simulink model "practika"  (R2024a)
settings: Solver=VariableStepAuto  StartTime=0.0  StopTime=15.0  RelTol=1e-3
model workspace (MAT data in the model file):
  diff_x = 0
  int_x = 0
  x = [1; 0]
  x1 = [-2; 0]
settings Model: Creator=Кирилл  LastModifiedBy=Анастасия
settings OptimizationCC: ReuseModelBlockBuffer=off
settings RTWCC: GPUComputeCapability=3.5

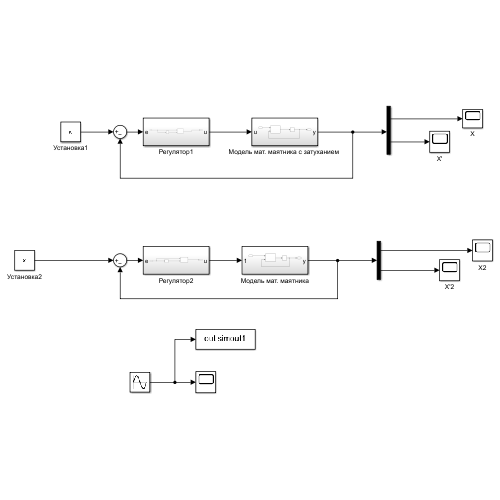
[thumbnail: Simulink's stored preview of the top-level diagram]
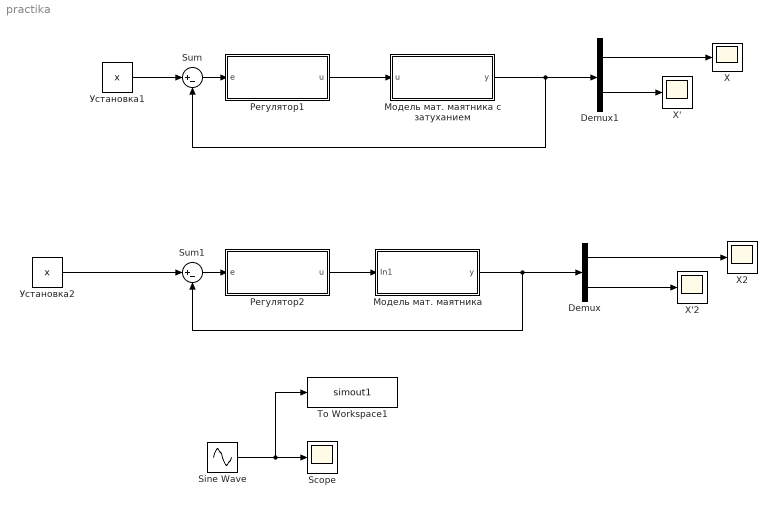
== system practika ==
  Demux : Demux  Outputs=2
  Demux1 : Demux  Outputs=2
  Scope : Scope
  Sine Wave : Sin  SampleTime=0
  Sum : Sum  Inputs=|+-
  Sum1 : Sum  Inputs=|+-
  To Workspace1 : ToWorkspace  VariableName=simout1  SaveFormat=Timeseries  SampleTime=-1
  X : Scope
  X' : Scope
  X'2 : Scope
  X2 : Scope
  Модель мат. маятника : Subsystem
  "Модель мат. маятника c затуханием " : Subsystem
  Регулятор1 : Subsystem
  Регулятор2 : Subsystem
  Установка1 : Constant  Value=x
  Установка2 : Constant  Value=x
  wires:
  Установка1/1 -> Sum/1
  "Модель мат. маятника c затуханием "/1(y) -> Sum/2, Demux1/1
  Sum/1 -> Регулятор1/1(e)
  Регулятор1/1(u) -> "Модель мат. маятника c затуханием "/1(u)
  Demux1/1 -> X/1
  Demux1/2 -> X'/1
  Установка2/1 -> Sum1/1
  Sum1/1 -> Регулятор2/1(e)
  Регулятор2/1(u) -> Модель мат. маятника/1(In1)
  Модель мат. маятника/1(y) -> Sum1/2, Demux/1
  Demux/1 -> X2/1
  Demux/2 -> X'2/1
  Sine Wave/1 -> To Workspace1/1, Scope/1

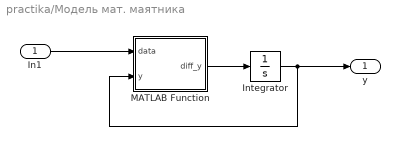
== system practika/Модель мат. маятника ==
  In1 : Inport
  Integrator : Integrator  InitialCondition=x1
  MATLAB Function : MATLAB Function  TreatAsAtomicUnit=on
  y : Outport
  wires:
  MATLAB Function/1(diff_y) -> Integrator/1
  Integrator/1 -> y/1, MATLAB Function/2(y)
  In1/1 -> MATLAB Function/1(data)

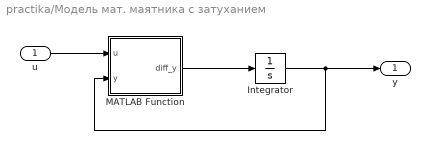
== system practika/Модель мат. маятника c затуханием  ==
  u : Inport
  Integrator : Integrator  InitialCondition=[-2;0]
  MATLAB Function : MATLAB Function  TreatAsAtomicUnit=on
  y : Outport
  wires:
  u/1 -> MATLAB Function/1(u)
  MATLAB Function/1(diff_y) -> Integrator/1
  Integrator/1 -> MATLAB Function/2(y), y/1

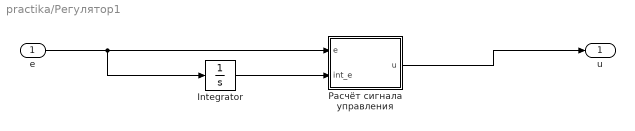
== system practika/Регулятор1 ==
  e : Inport
  Integrator : Integrator
  Расчёт сигнала управления : MATLAB Function  TreatAsAtomicUnit=on
  u : Outport
  wires:
  e/1 -> Расчёт сигнала управления/1(e), Integrator/1
  Integrator/1 -> Расчёт сигнала управления/2(int_e)
  Расчёт сигнала управления/1(u) -> u/1

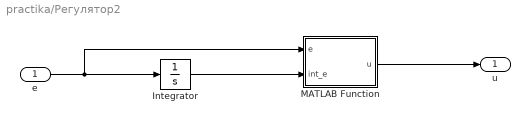
== system practika/Регулятор2 ==
  e : Inport
  Integrator : Integrator
  MATLAB Function : MATLAB Function  TreatAsAtomicUnit=on
  u : Outport
  wires:
  e/1 -> MATLAB Function/1(e), Integrator/1
  Integrator/1 -> MATLAB Function/2(int_e)
  MATLAB Function/1(u) -> u/1

== matlab function practika/Модель мат. маятника c затуханием /MATLAB Function ==
  data: u input; diff_y output; y input
function diff_y = fcn(u, y)

g = 9.81;
m = 0.5;
b = 1;
c = 1;
l = 0.1;
% diff_y = zeros(1,2);
% 
% diff_y(1, 1) =  y(2);
% diff_y(1, 2) = -(g/l)*sin(y(1)) - (b*y(2))/(m*(l^2)) - c*y(1)/(m*(l^2)) + u/(m*(l^2));
diff_y=[y(2); -(g/l)*sin(y(1)) - (b*y(2))/(m*(l^2)) - c*y(1)/(m*(l^2)) + u/(m*(l^2)) ];
end

== matlab function practika/Регулятор1/Расчёт сигнала управления ==
  data: e input; int_e input; u output
function u = fcn(e, int_e)
Kp = 2;
K1 = 2;


u = Kp*e(1) + Kp*e(2) + K1*int_e(1) + K1*int_e(2);
end

== matlab function practika/Модель мат. маятника/MATLAB Function ==
  data: data input; diff_y output; y input
function diff_y = fcn(data, y)

    g = 9.81;
    l = 0.1;
    m = 0.5;

    % diff_y(1, 2) = -(g/l)*sin(y(1)) - (b*y(2))/(m*(l^2)) - c*y(1)/(m*(l^2)) + u/(m*(l^2));

    diff_y=[y(2); -(g/l)*sin(y(1))];

end

== matlab function practika/Регулятор2/MATLAB Function ==
  data: e input; int_e input; u output
function u = fcn(e, int_e)

    K1 = 2;
    K2 = 0.5;
    
    u=K1*e(1)+K1*e(2)+K2*int_e(1)+K2*int_e(2);
    
end
